simulink model "for_loop"  (R2022b)
settings: Solver=FixedStepAuto  StartTime=0.0  StopTime=5  FixedStep=1  RelTol=1e-3
settings Model: Creator=Dell  LastModifiedBy=Dell

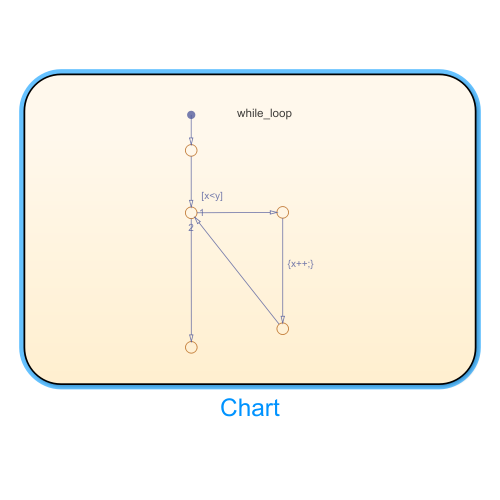
[thumbnail: Simulink's stored preview of the top-level diagram]
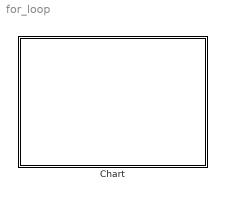
== system for_loop ==
  Chart : Stateflow chart  TreatAsAtomicUnit=on

== stateflow chart for_loop/Chart ==
  note: while_loop
  (default) -> (junction 197)
  (junction 197) -> (junction 199)
  (junction 199) -> (junction 198) [order 1] : [x<y]
  (junction 200) -> (junction 199)
  (junction 198) -> (junction 200) : {x++;}
  (junction 199) -> (junction 201) [order 2]
  data: y local int8 =5; x local int8 =0
